simulink model "ej2"  (R2023a)
settings: Solver=VariableStepAuto  StartTime=0.0  StopTime=70  MaxStep=1e-4  RelTol=1e-3
libraries: SignalEditorBlockLib x6
settings Model: Creator=Juan  LastModifiedBy=Juan

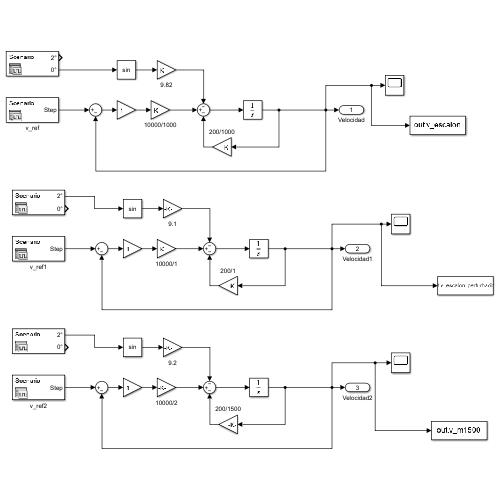
[thumbnail: Simulink's stored preview of the top-level diagram]
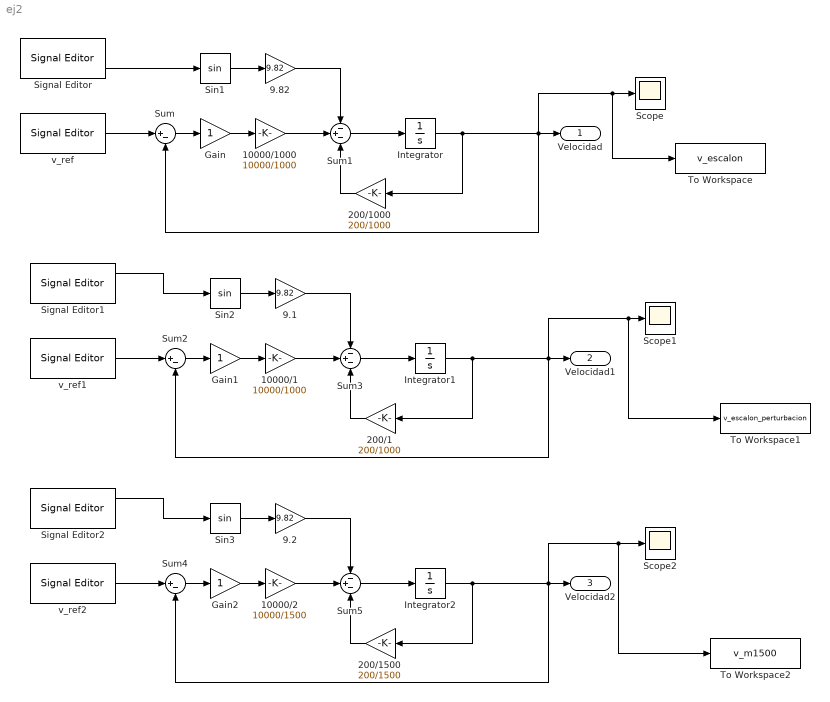
== system ej2 ==
  10000/1 : Gain  Gain=10000/1000
  10000/1000 : Gain  Gain=10000/1000
  10000/2 : Gain  Gain=10000/1500
  200/1 : Gain  Gain=200/1000
  200/1000 : Gain  Gain=200/1000
  200/1500 : Gain  Gain=200/1500
  9.1 : Gain  Gain=9.82
  9.2 : Gain  Gain=9.82
  9.82 : Gain  Gain=9.82
  Gain : Gain
  Gain1 : Gain
  Gain2 : Gain
  Integrator : Integrator  InitialCondition=25
  Integrator1 : Integrator  InitialCondition=25
  Integrator2 : Integrator  InitialCondition=25
  Scope : Scope
  Scope1 : Scope
  Scope2 : Scope
  Signal Editor : SignalEditorBlockLib/Signal Editor  FileName=perturbn.mat  ActiveScenario=Scenario  ActiveSignal=2°  IsBus=off  OutputBusObjectStr=Bus: BusObject  SampleTime=0  Interpolate=off  ZeroCross=off  OutputAfterFinalValue=Setting to zero  Unit=inherit  PreserveSignalName=on  ApplySigPropsToAllScenarios=on
  Signal Editor1 : SignalEditorBlockLib/Signal Editor  FileName=perturbn.mat  ActiveScenario=Scenario  ActiveSignal=2°  IsBus=off  OutputBusObjectStr=Bus: BusObject  SampleTime=0  Interpolate=off  ZeroCross=off  OutputAfterFinalValue=Setting to zero  Unit=inherit  PreserveSignalName=on  ApplySigPropsToAllScenarios=on
  Signal Editor2 : SignalEditorBlockLib/Signal Editor  FileName=perturbn.mat  ActiveScenario=Scenario  ActiveSignal=2°  IsBus=off  OutputBusObjectStr=Bus: BusObject  SampleTime=0  Interpolate=off  ZeroCross=off  OutputAfterFinalValue=Setting to zero  Unit=inherit  PreserveSignalName=on  ApplySigPropsToAllScenarios=on
  Sin1 : Trigonometry
  Sin2 : Trigonometry
  Sin3 : Trigonometry
  Sum : Sum  Inputs=|+-
  Sum1 : Sum  Inputs=-+-
  Sum2 : Sum  Inputs=|+-
  Sum3 : Sum  Inputs=-+-
  Sum4 : Sum  Inputs=|+-
  Sum5 : Sum  Inputs=-+-
  To Workspace : ToWorkspace  VariableName=v_escalon  SaveFormat=Timeseries  SampleTime=-1
  To Workspace1 : ToWorkspace  VariableName=v_escalon_perturbacion  SaveFormat=Timeseries  SampleTime=-1
  To Workspace2 : ToWorkspace  VariableName=v_m1500  SaveFormat=Timeseries  SampleTime=-1
  v_ref : SignalEditorBlockLib/Signal Editor  FileName=v_ref.mat  ActiveScenario=Scenario  ActiveSignal=Step  IsBus=off  OutputBusObjectStr=Bus: BusObject  SampleTime=0  Interpolate=off  ZeroCross=off  OutputAfterFinalValue=Setting to zero  Unit=inherit  PreserveSignalName=on  ApplySigPropsToAllScenarios=on
  v_ref1 : SignalEditorBlockLib/Signal Editor  FileName=v_ref.mat  ActiveScenario=Scenario  ActiveSignal=Step  IsBus=off  OutputBusObjectStr=Bus: BusObject  SampleTime=0  Interpolate=off  ZeroCross=off  OutputAfterFinalValue=Setting to zero  Unit=inherit  PreserveSignalName=on  ApplySigPropsToAllScenarios=on
  v_ref2 : SignalEditorBlockLib/Signal Editor  FileName=v_ref.mat  ActiveScenario=Scenario  ActiveSignal=Step  IsBus=off  OutputBusObjectStr=Bus: BusObject  SampleTime=0  Interpolate=off  ZeroCross=off  OutputAfterFinalValue=Setting to zero  Unit=inherit  PreserveSignalName=on  ApplySigPropsToAllScenarios=on
  Velocidad : Outport
  Velocidad1 : Outport  Port=2
  Velocidad2 : Outport  Port=3
  wires:
  v_ref/1 -> Sum/1
  Signal Editor/2 -> Sin1/1
  Sin1/1 -> 9.82/1
  9.82/1 -> Sum1/1
  200/1000/1 -> Sum1/3
  Sum1/1 -> Integrator/1
  Integrator/1 -> 200/1000/1, Sum/2, To Workspace/1, Scope/1, Velocidad/1
  Sum/1 -> Gain/1
  Gain/1 -> 10000/1000/1
  10000/1000/1 -> Sum1/2
  Sin2/1 -> 9.1/1
  Sum3/1 -> Integrator1/1
  9.1/1 -> Sum3/1
  v_ref1/1 -> Sum2/1
  Gain1/1 -> 10000/1/1
  Sum2/1 -> Gain1/1
  10000/1/1 -> Sum3/2
  Signal Editor1/1 -> Sin2/1
  200/1/1 -> Sum3/3
  9.2/1 -> Sum5/1
  Sin3/1 -> 9.2/1
  Sum5/1 -> Integrator2/1
  200/1500/1 -> Sum5/3
  Signal Editor2/1 -> Sin3/1
  10000/2/1 -> Sum5/2
  Sum4/1 -> Gain2/1
  v_ref2/1 -> Sum4/1
  Gain2/1 -> 10000/2/1
  Integrator1/1 -> 200/1/1, Sum2/2, To Workspace1/1, Scope1/1, Velocidad1/1
  Integrator2/1 -> 200/1500/1, Sum4/2, To Workspace2/1, Scope2/1, Velocidad2/1
